simulink model "Compare"  (R2016b)
settings: Solver=VariableStepAuto  StartTime=0.0  StopTime=10.0  RelTol=1e-3
values from neighbouring files (symbols this model uses):
  b = [-0.00316056348294 0.00600370510414 0.0345483654264 0.0245303741972 -0.0579381144345 -0.06741428459 0.153841471553 0.436190208002 0.436190208002 0.153841471553 -0.06741428459 -0.0579381144345 ... (16 elements, 1x16)]    [firworkspace.mat]
libraries: dspstat3 x4, dspsrcs4 x2
settings Model: FPTRunName=Initial_FP  Creator=user  LastModifiedBy=user
settings DebuggingCC: SignalRangeChecking=warning  ParameterDowncastMsg=warning  ParameterOverflowMsg=warning

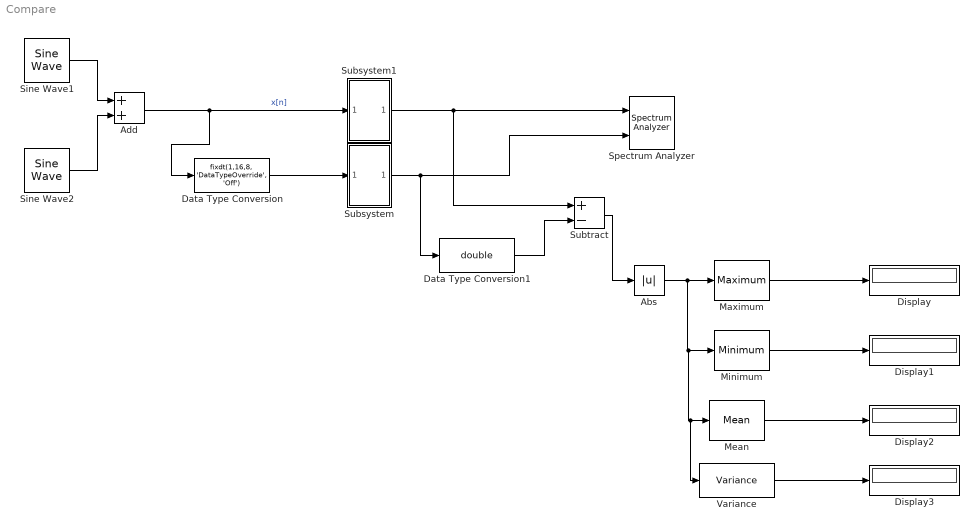
== system Compare ==
  Abs : Abs
  Add : Sum
  Data Type Conversion : DataTypeConversion  OutDataTypeStr=fixdt(1,16,8, 'DataTypeOverride', 'Off')
  Data Type Conversion1 : DataTypeConversion  OutDataTypeStr=double
  Display{,1..3} (4 alike) : Display
  Maximum : dspstat3/Maximum  operation=maximum  fcn=Running  indexBase=One  operateOver=Each column  Dimension=1  reset=None  roiEnable=off  roiType=Rectangles  roiPortion=Entire ROI  roiOutput=Individual statistics for each ROI  roiFlag=off  roundingMode=Floor  overflowMode=off  accumDataTypeStr=Inherit: Same as product output  accumLastDataTypeStr=Inherit: Same as product output
  Mean : dspstat3/Mean  run=on  reset_popup=None  directionMode=Each column  dimension=1  roiEnable=off  roiType=Rectangles  roiPortion=Entire ROI  roiOutput=Individual statistics for each ROI  roiFlag=off  outputDataTypeStr=Inherit: Same as accumulator  outputLastDataTypeStr=Inherit: Same as accumulator  outputMin=[]  outputMax=[]  roundingMode=Floor  overflowMode=off
  Minimum : dspstat3/Minimum  operation=minimum  fcn=Running  indexBase=One  operateOver=Entire input  Dimension=1  reset=None  roiEnable=off  roiType=Rectangles  roiPortion=Entire ROI  roiOutput=Individual statistics for each ROI  roiFlag=off  roundingMode=Floor  overflowMode=off
  Sine Wave1 : dspsrcs4/Sine Wave  Amplitude=28  Frequency=4000  Phase=0  SampleMode=Discrete  OutComplex=Real  CompMethod=Trigonometric fcn  TableSize=Speed  SampleTime=1/42000  SamplesPerFrame=1  ResetState=Restart at time zero  OutputFrames=off  dataType=double  wordLen=16  udDataType=sfix(16)  fracBitsMode=Best precision  numFracBits=15  OutDataTypeStr=double  LastOutDataTypeStr=double
  Sine Wave2 : dspsrcs4/Sine Wave  Amplitude=66  Frequency=17500  Phase=0  SampleMode=Discrete  OutComplex=Real  CompMethod=Trigonometric fcn  TableSize=Speed  SampleTime=1/42000  SamplesPerFrame=1  ResetState=Restart at time zero  OutputFrames=off  dataType=double  wordLen=16  udDataType=sfix(16)  fracBitsMode=Best precision  numFracBits=15  OutDataTypeStr=double  LastOutDataTypeStr=double
  Spectrum Analyzer : SpectrumAnalyzer  NumInputPorts=2
  Subsystem : Subsystem  MinMaxOverflowLogging=MinMaxAndOverflow
  Subsystem1 : Subsystem
  Subtract : Sum  Inputs=+-
  Variance : dspstat3/Variance  run=on  reset_popup=None  directionMode=Each column  dimension=1  roiEnable=off  roiType=Rectangles  roiPortion=Entire ROI  roiOutput=Individual statistics for each ROI  roiFlag=off  roundingMode=Floor  overflowMode=off
  wires:
  Add/1 -> Data Type Conversion/1, Subsystem1/1(In1)  "x[n]"
  Subsystem/1(Out1) -> Data Type Conversion1/1, Spectrum Analyzer/2
  Sine Wave2/1 -> Add/2
  Sine Wave1/1 -> Add/1
  Data Type Conversion/1 -> Subsystem/1(In1)
  Subsystem1/1(Out1) -> Subtract/1, Spectrum Analyzer/1
  Subtract/1 -> Abs/1
  Data Type Conversion1/1 -> Subtract/2
  Abs/1 -> Maximum/1, Minimum/1, Variance/1, Mean/1
  Variance/1 -> Display3/1
  Mean/1 -> Display2/1
  Minimum/1 -> Display1/1
  Maximum/1 -> Display/1

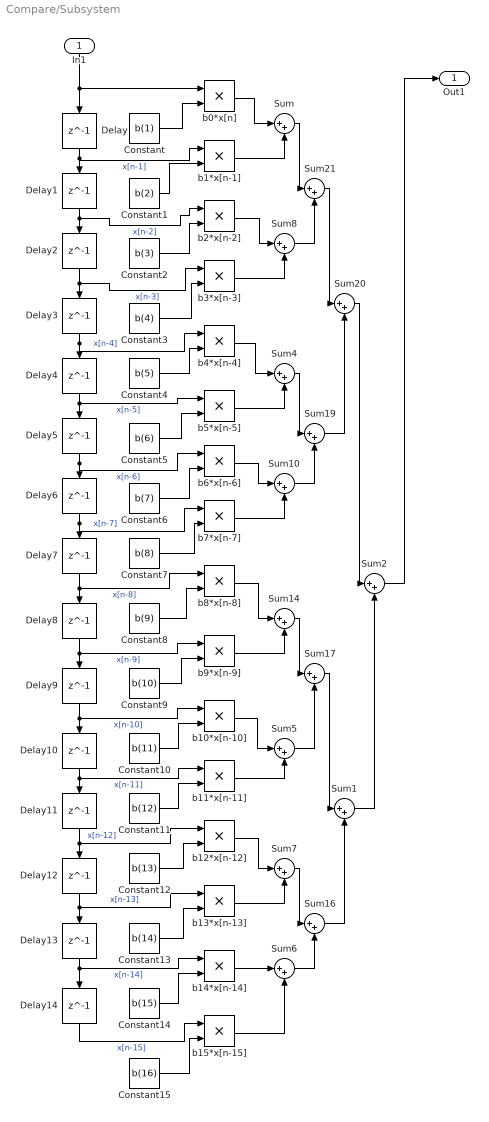
== system Compare/Subsystem ==
  In1 : Inport  OutMin=-94  OutMax=94  OutDataTypeStr=fixdt(1,16,8)
  Constant : Constant  Value=b(1)  OutDataTypeStr=fixdt(1,16,23)
  Constant1 : Constant  Value=b(2)  OutDataTypeStr=fixdt(0,16,23)
  Constant10 : Constant  Value=b(11)  OutDataTypeStr=fixdt(1,16,18)
  Constant11 : Constant  Value=b(12)  OutDataTypeStr=fixdt(1,16,19)
  Constant12 : Constant  Value=b(13)  OutDataTypeStr=fixdt(0,16,21)
  Constant13 : Constant  Value=b(14)  OutDataTypeStr=fixdt(0,16,20)
  Constant14 : Constant  Value=b(15)  OutDataTypeStr=fixdt(0,16,23)
  Constant15 : Constant  Value=b(16)  OutDataTypeStr=fixdt(1,16,23)
  Constant2 : Constant  Value=b(3)  OutDataTypeStr=fixdt(0,16,20)
  Constant3 : Constant  Value=b(4)  OutDataTypeStr=fixdt(0,16,21)
  Constant4 : Constant  Value=b(5)  OutDataTypeStr=fixdt(1,16,19)
  Constant5 : Constant  Value=b(6)  OutDataTypeStr=fixdt(1,16,18)
  Constant6 : Constant  Value=b(7)  OutDataTypeStr=fixdt(0,16,18)
  Constant7 : Constant  Value=b(8)  OutDataTypeStr=fixdt(0,16,17)
  Constant8 : Constant  Value=b(9)  OutDataTypeStr=fixdt(0,16,17)
  Constant9 : Constant  Value=b(10)  OutDataTypeStr=fixdt(0,16,18)
  Delay{,1..14} (15 alike) : Delay  DelayLength=1  InitialCondition=0
  Sum : Sum  Inputs=|++  OutDataTypeStr=fixdt(1,16,15)
  Sum{1,10,14,17,19..20} (6 alike) : Sum  Inputs=|++  OutDataTypeStr=fixdt(1,16,9)
  Sum{7..8,16,21} (4 alike) : Sum  Inputs=|++  OutDataTypeStr=fixdt(1,16,13)
  Sum2 : Sum  Inputs=|++  OutDataTypeStr=fixdt(1,16,10)
  Sum4 : Sum  Inputs=|++  OutDataTypeStr=fixdt(1,16,12)
  Sum5 : Sum  Inputs=|++  OutDataTypeStr=fixdt(1,16,12)
  Sum6 : Sum  Inputs=|++  OutDataTypeStr=fixdt(1,16,15)
  b0*x[n] : Product  OutDataTypeStr=fixdt(1,16,16)
  b1*x[n-1] : Product  OutDataTypeStr=fixdt(1,16,15)
  b10*x[n-10] : Product  OutDataTypeStr=fixdt(1,16,12)
  b11*x[n-11] : Product  OutDataTypeStr=fixdt(1,16,12)
  b12*x[n-12] : Product  OutDataTypeStr=fixdt(1,16,13)
  b13*x[n-13] : Product  OutDataTypeStr=fixdt(1,16,13)
  b14*x[n-14] : Product  OutDataTypeStr=fixdt(1,16,15)
  b15*x[n-15] : Product  OutDataTypeStr=fixdt(1,16,16)
  b2*x[n-2] : Product  OutDataTypeStr=fixdt(1,16,13)
  b3*x[n-3] : Product  OutDataTypeStr=fixdt(1,16,13)
  b4*x[n-4] : Product  OutDataTypeStr=fixdt(1,16,12)
  b5*x[n-5] : Product  OutDataTypeStr=fixdt(1,16,12)
  b6*x[n-6] : Product  OutDataTypeStr=fixdt(1,16,11)
  b7*x[n-7] : Product  OutDataTypeStr=fixdt(1,16,9)
  b8*x[n-8] : Product  OutDataTypeStr=fixdt(1,16,9)
  b9*x[n-9] : Product  OutDataTypeStr=fixdt(1,16,11)
  Out1 : Outport
  wires:
  b13*x[n-13]/1 -> Sum7/2
  b11*x[n-11]/1 -> Sum5/2
  b15*x[n-15]/1 -> Sum6/2
  b14*x[n-14]/1 -> Sum6/1
  b4*x[n-4]/1 -> Sum4/1
  Delay4/1 -> b5*x[n-5]/1, Delay5/1  "x[n-5]"
  b3*x[n-3]/1 -> Sum8/2
  Sum19/1 -> Sum20/2
  Sum1/1 -> Sum2/2
  b0*x[n]/1 -> Sum/1
  In1/1 -> b0*x[n]/1, Delay/1
  b9*x[n-9]/1 -> Sum14/2
  b12*x[n-12]/1 -> Sum7/1
  b7*x[n-7]/1 -> Sum10/2
  b1*x[n-1]/1 -> Sum/2
  b6*x[n-6]/1 -> Sum10/1
  Sum17/1 -> Sum1/1
  Sum7/1 -> Sum16/1
  b8*x[n-8]/1 -> Sum14/1
  Sum10/1 -> Sum19/2
  b2*x[n-2]/1 -> Sum8/1
  Sum14/1 -> Sum17/1
  Sum16/1 -> Sum1/2
  Sum8/1 -> Sum21/2
  b5*x[n-5]/1 -> Sum4/2
  Sum6/1 -> Sum16/2
  Sum/1 -> Sum21/1
  Sum4/1 -> Sum19/1
  Sum5/1 -> Sum17/2
  Sum21/1 -> Sum20/1
  Sum2/1 -> Out1/1
  b10*x[n-10]/1 -> Sum5/1
  Sum20/1 -> Sum2/1
  Delay10/1 -> b11*x[n-11]/1, Delay11/1  "x[n-11]"
  Delay5/1 -> b6*x[n-6]/1, Delay6/1  "x[n-6]"
  Delay14/1 -> b15*x[n-15]/1  "x[n-15]"
  Delay13/1 -> b14*x[n-14]/1, Delay14/1  "x[n-14]"
  Delay9/1 -> b10*x[n-10]/1, Delay10/1  "x[n-10]"
  Delay/1 -> Delay1/1, b1*x[n-1]/1  "x[n-1]"
  Delay1/1 -> b2*x[n-2]/1, Delay2/1  "x[n-2]"
  Delay11/1 -> b12*x[n-12]/1, Delay12/1  "x[n-12]"
  Delay8/1 -> b9*x[n-9]/1, Delay9/1  "x[n-9]"
  Delay6/1 -> b7*x[n-7]/1, Delay7/1  "x[n-7]"
  Delay12/1 -> b13*x[n-13]/1, Delay13/1  "x[n-13]"
  Delay3/1 -> b4*x[n-4]/1, Delay4/1  "x[n-4]"
  Delay2/1 -> b3*x[n-3]/1, Delay3/1  "x[n-3]"
  Delay7/1 -> b8*x[n-8]/1, Delay8/1  "x[n-8]"
  Constant/1 -> b0*x[n]/2
  Constant1/1 -> b1*x[n-1]/2
  Constant2/1 -> b2*x[n-2]/2
  Constant3/1 -> b3*x[n-3]/2
  Constant4/1 -> b4*x[n-4]/2
  Constant5/1 -> b5*x[n-5]/2
  Constant6/1 -> b6*x[n-6]/2
  Constant7/1 -> b7*x[n-7]/2
  Constant8/1 -> b8*x[n-8]/2
  Constant9/1 -> b9*x[n-9]/2
  Constant10/1 -> b10*x[n-10]/2
  Constant11/1 -> b11*x[n-11]/2
  Constant12/1 -> b12*x[n-12]/2
  Constant13/1 -> b13*x[n-13]/2
  Constant14/1 -> b14*x[n-14]/2
  Constant15/1 -> b15*x[n-15]/2

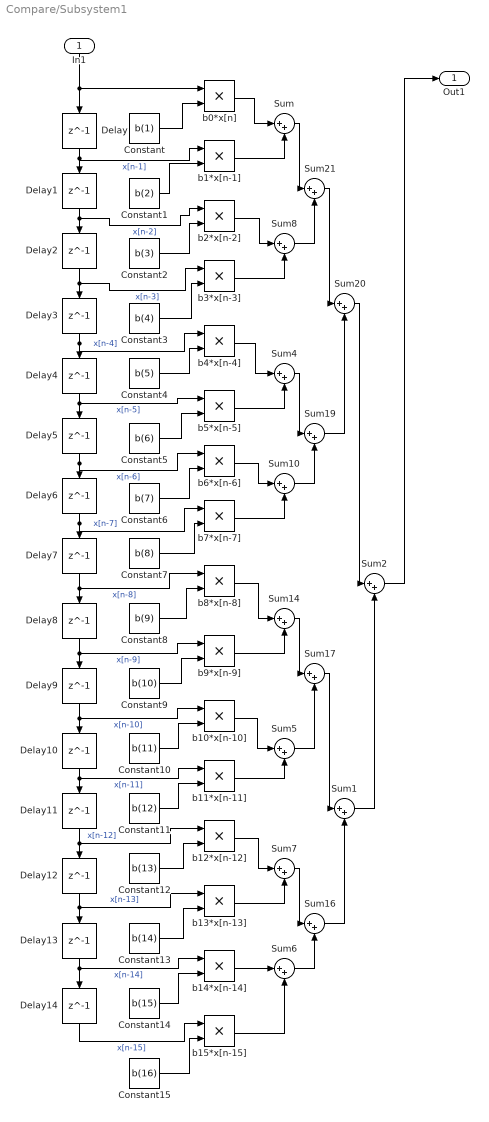
== system Compare/Subsystem1 ==
  In1 : Inport
  Constant : Constant  Value=b(1)
  Constant1 : Constant  Value=b(2)
  Constant10 : Constant  Value=b(11)
  Constant11 : Constant  Value=b(12)
  Constant12 : Constant  Value=b(13)
  Constant13 : Constant  Value=b(14)
  Constant14 : Constant  Value=b(15)
  Constant15 : Constant  Value=b(16)
  Constant2 : Constant  Value=b(3)
  Constant3 : Constant  Value=b(4)
  Constant4 : Constant  Value=b(5)
  Constant5 : Constant  Value=b(6)
  Constant6 : Constant  Value=b(7)
  Constant7 : Constant  Value=b(8)
  Constant8 : Constant  Value=b(9)
  Constant9 : Constant  Value=b(10)
  Delay{,1..14} (15 alike) : Delay  DelayLength=1  InitialCondition=0
  Sum{,1..2,4..8,10,14,16..17,19..21} (15 alike) : Sum  Inputs=|++
  b0*x[n] : Product
  b1*x[n-1] : Product
  b10*x[n-10] : Product
  b11*x[n-11] : Product
  b12*x[n-12] : Product
  b13*x[n-13] : Product
  b14*x[n-14] : Product
  b15*x[n-15] : Product
  b2*x[n-2] : Product
  b3*x[n-3] : Product
  b4*x[n-4] : Product
  b5*x[n-5] : Product
  b6*x[n-6] : Product
  b7*x[n-7] : Product
  b8*x[n-8] : Product
  b9*x[n-9] : Product
  Out1 : Outport
  wires:
  b13*x[n-13]/1 -> Sum7/2
  b11*x[n-11]/1 -> Sum5/2
  b15*x[n-15]/1 -> Sum6/2
  b14*x[n-14]/1 -> Sum6/1
  b4*x[n-4]/1 -> Sum4/1
  Delay4/1 -> b5*x[n-5]/1, Delay5/1  "x[n-5]"
  b3*x[n-3]/1 -> Sum8/2
  Sum19/1 -> Sum20/2
  Sum1/1 -> Sum2/2
  b0*x[n]/1 -> Sum/1
  In1/1 -> b0*x[n]/1, Delay/1
  b9*x[n-9]/1 -> Sum14/2
  b12*x[n-12]/1 -> Sum7/1
  b7*x[n-7]/1 -> Sum10/2
  b1*x[n-1]/1 -> Sum/2
  b6*x[n-6]/1 -> Sum10/1
  Sum17/1 -> Sum1/1
  Sum7/1 -> Sum16/1
  b8*x[n-8]/1 -> Sum14/1
  Sum10/1 -> Sum19/2
  b2*x[n-2]/1 -> Sum8/1
  Sum14/1 -> Sum17/1
  Sum16/1 -> Sum1/2
  Sum8/1 -> Sum21/2
  b5*x[n-5]/1 -> Sum4/2
  Sum6/1 -> Sum16/2
  Sum/1 -> Sum21/1
  Sum4/1 -> Sum19/1
  Sum5/1 -> Sum17/2
  Sum21/1 -> Sum20/1
  Sum2/1 -> Out1/1
  b10*x[n-10]/1 -> Sum5/1
  Sum20/1 -> Sum2/1
  Delay10/1 -> b11*x[n-11]/1, Delay11/1  "x[n-11]"
  Delay5/1 -> b6*x[n-6]/1, Delay6/1  "x[n-6]"
  Delay14/1 -> b15*x[n-15]/1  "x[n-15]"
  Delay13/1 -> b14*x[n-14]/1, Delay14/1  "x[n-14]"
  Delay9/1 -> b10*x[n-10]/1, Delay10/1  "x[n-10]"
  Delay/1 -> Delay1/1, b1*x[n-1]/1  "x[n-1]"
  Delay1/1 -> b2*x[n-2]/1, Delay2/1  "x[n-2]"
  Delay11/1 -> b12*x[n-12]/1, Delay12/1  "x[n-12]"
  Delay8/1 -> b9*x[n-9]/1, Delay9/1  "x[n-9]"
  Delay6/1 -> b7*x[n-7]/1, Delay7/1  "x[n-7]"
  Delay12/1 -> b13*x[n-13]/1, Delay13/1  "x[n-13]"
  Delay3/1 -> b4*x[n-4]/1, Delay4/1  "x[n-4]"
  Delay2/1 -> b3*x[n-3]/1, Delay3/1  "x[n-3]"
  Delay7/1 -> b8*x[n-8]/1, Delay8/1  "x[n-8]"
  Constant/1 -> b0*x[n]/2
  Constant1/1 -> b1*x[n-1]/2
  Constant2/1 -> b2*x[n-2]/2
  Constant3/1 -> b3*x[n-3]/2
  Constant4/1 -> b4*x[n-4]/2
  Constant5/1 -> b5*x[n-5]/2
  Constant6/1 -> b6*x[n-6]/2
  Constant7/1 -> b7*x[n-7]/2
  Constant8/1 -> b8*x[n-8]/2
  Constant9/1 -> b9*x[n-9]/2
  Constant10/1 -> b10*x[n-10]/2
  Constant11/1 -> b11*x[n-11]/2
  Constant12/1 -> b12*x[n-12]/2
  Constant13/1 -> b13*x[n-13]/2
  Constant14/1 -> b14*x[n-14]/2
  Constant15/1 -> b15*x[n-15]/2
